simulink model "quadcopter_mpc_position_test"  (R2015b)
settings: Solver=VariableStepAuto  StartTime=0.0  StopTime=50  FixedStep=0.2  RelTol=1e-3
undefined symbols (not defined in the file): md_quadcopter, seed
libraries: vrlib x2
settings Model: Creator=Daniel  LastModifiedBy=mgreiff
settings SolverCC: AlgebraicLoopSolver=LineSearch

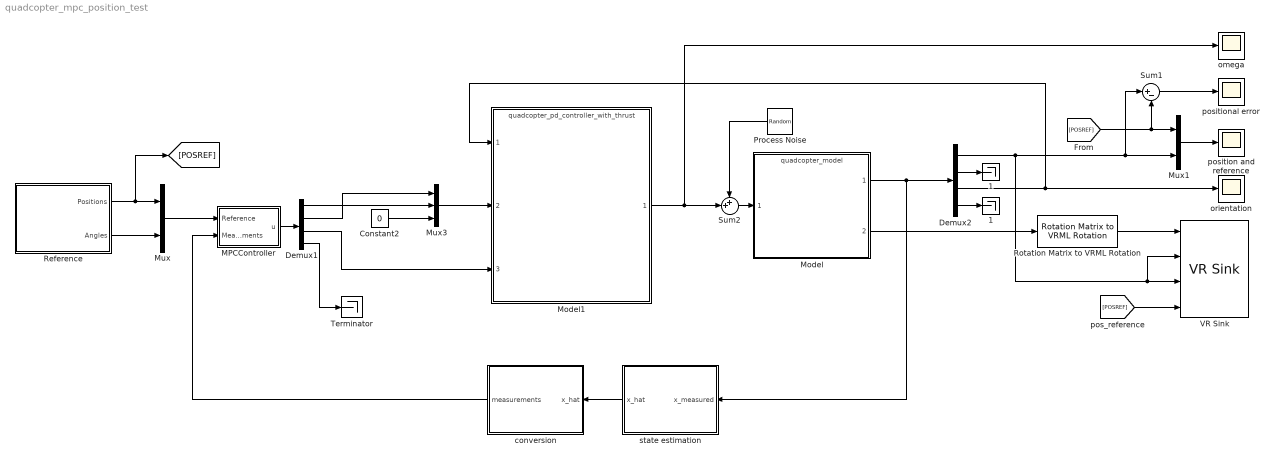
== system quadcopter_mpc_position_test ==
  "   1" : Terminator
  "  1" : Terminator
  Constant2 : Constant  Value=0
  Demux1 : Demux
  Demux2 : Demux  Outputs=[3,3,3,3]
  MPCController : Subsystem  mask{md=md_quadcopter}
      mask prompts: md "MPCData"
  Model : ModelReference  ModelNameDialog=quadcopter_model.mdl  SimulationMode=Normal  ModelReferenceVersion=1.117  CopyOfModelName=quadcopter_model.mdl
  Model1 : ModelReference  ModelNameDialog=quadcopter_pd_controller_with_thrust.mdl  SimulationMode=Normal  ModelReferenceVersion=1.70  CopyOfModelName=quadcopter_pd_controller_with_thrust.mdl
  Mux : Mux  Inputs=2
  Mux1 : Mux  Inputs=2
  Mux3 : Mux  Inputs=3
  Process Noise : RandomNumber  Mean=[0 0 0 0]'  Variance=0  SampleTime=0.2
  Reference : Subsystem
  Rotation Matrix to VRML Rotation : vrlib/Utilities/Rotation Matrix to VRML Rotation  maxzero=1e-12
  Sum1 : Sum  Inputs=|+-
  Sum2 : Sum  Inputs=++|
  Terminator : Terminator
  VR Sink : vrlib/VR Sink  InstantiateOnLoad=on  SampleTime=0.05  ViewEnable=on  RemoteChange=off  RemoteView=off  FieldsWritten=copter.rotation.4.1.1.double#copter.translation.3.1.1.double#vp.translation.3.1.1.double#target.translation.3.1.1.double  WorldFileName=copter_world.wrl  WorldDescription=quadcopter_world  AutoView=on  VideoDimensions=[]  AllowVariableSize=off
  conversion : Subsystem
  "omega " : Scope
  orientation : Scope
  position and reference : Scope
  positional error : Scope
  state estimation : Subsystem
  wires:
  Model/2 -> Rotation Matrix to VRML Rotation/1
  Rotation Matrix to VRML Rotation/1 -> VR Sink/1
  Process Noise/1 -> Sum2/1
  Mux/1 -> MPCController/1(Reference)
  MPCController/1(u) -> Demux1/1
  Demux1/3 -> Model1/3
  Mux3/1 -> Model1/2
  Constant2/1 -> Mux3/3
  Demux1/2 -> Mux3/1
  Demux1/1 -> Mux3/2
  Sum2/1 -> Model/1
  Demux1/4 -> Terminator/1
  Reference/2(Angles) -> Mux/2
  [POSREF] -> VR Sink/4
  conversion/1(measurements) -> MPCController/2(Measurements)
  Model1/1 -> "omega "/1, Sum2/2
  [POSREF] -> Sum1/2, Mux1/1
  Mux1/1 -> position and reference/1
  Sum1/1 -> positional error/1
  Demux2/1 -> VR Sink/2, VR Sink/3, Sum1/1, Mux1/2
  Demux2/2 -> "  1"/1
  Demux2/4 -> "   1"/1
  Demux2/3 -> Model1/1, orientation/1
  Model/1 -> state estimation/1(x_measured), Demux2/1
  state estimation/1(x_hat) -> conversion/1(x_hat)
  Reference/1(Positions) -> [POSREF], Mux/1

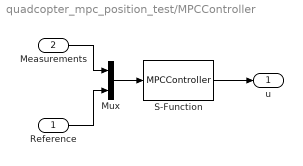
== system quadcopter_mpc_position_test/MPCController ==
  Reference : Inport
  Measurements : Inport  Port=2
  Mux : Mux  Inputs=2
  S-Function : S-Function  FunctionName=MPCController  Parameters=md  SFunctionDeploymentMode=off  EnableBusSupport=off
  u : Outport
  wires:
  S-Function/1 -> u/1
  Reference/1 -> Mux/2
  Measurements/1 -> Mux/1
  Mux/1 -> S-Function/1

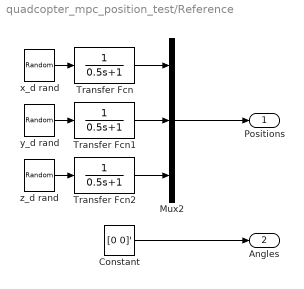
== system quadcopter_mpc_position_test/Reference ==
  Constant : Constant  Value=[0 0]'  SampleTime=10
  Mux2 : Mux  Inputs=3
  Transfer Fcn : TransferFcn  Denominator=[0.5 1]
  Transfer Fcn1 : TransferFcn  Denominator=[0.5 1]
  Transfer Fcn2 : TransferFcn  Denominator=[0.5 1]
  x_d rand : UniformRandomNumber  Minimum=-30  Maximum=30  Seed=0+seed  SampleTime=10
  y_d rand : UniformRandomNumber  Minimum=-30  Maximum=30  Seed=1+seed  SampleTime=10
  z_d rand : UniformRandomNumber  Minimum=0  Maximum=15  Seed=2+seed  SampleTime=10
  Positions : Outport
  Angles : Outport  Port=2
  wires:
  x_d rand/1 -> Transfer Fcn/1
  y_d rand/1 -> Transfer Fcn1/1
  z_d rand/1 -> Transfer Fcn2/1
  Transfer Fcn/1 -> Mux2/1
  Transfer Fcn1/1 -> Mux2/2
  Transfer Fcn2/1 -> Mux2/3
  Constant/1 -> Angles/1
  Mux2/1 -> Positions/1

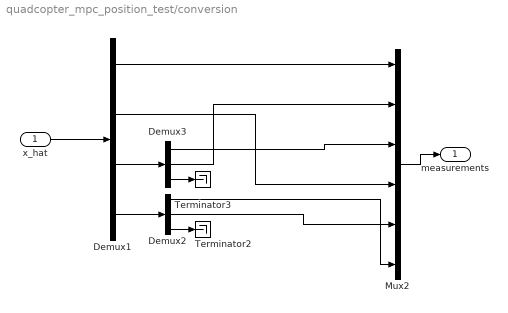
== system quadcopter_mpc_position_test/conversion ==
  x_hat : Inport
  Demux1 : Demux  Outputs=[3,3,3,3]
  Demux2 : Demux  Outputs=3
  Demux3 : Demux  Outputs=3
  Mux2 : Mux  Inputs=6
  Terminator2 : Terminator
  Terminator3 : Terminator
  measurements : Outport
  wires:
  Mux2/1 -> measurements/1
  x_hat/1 -> Demux1/1
  Demux1/1 -> Mux2/1
  Demux1/2 -> Mux2/4
  Demux2/3 -> Terminator2/1
  Demux1/4 -> Demux2/1
  Demux3/3 -> Terminator3/1
  Demux1/3 -> Demux3/1
  Demux3/2 -> Mux2/2
  Demux3/1 -> Mux2/3
  Demux2/1 -> Mux2/6
  Demux2/2 -> Mux2/5

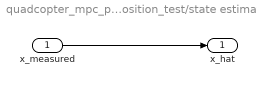
== system quadcopter_mpc_position_test/state estimation ==
  x_measured : Inport
  x_hat : Outport
  wires:
  x_measured/1 -> x_hat/1
